simulink model "Vergleich_MRAC"  (Simulink 7.8)
settings: Solver=ode45  StartTime=0.0  StopTime=40  MaxStep=1e-4  RelTol=1e-4
values from neighbouring files (symbols this model uses):
  A = [0,1;-0.4,-0.5]    [Vergleich_MRAC_L1.m]
  Am = [0,1;-2,-2]    [Vergleich_MRAC_L1.m]
  b = [0;1]    [Vergleich_MRAC_L1.m]
  c = [1,0]    [Vergleich_MRAC_L1.m]
  cm = [1,0]    [Vergleich_MRAC_L1.m]
  Gamma2 = 10    [Vergleich_MRAC_L1.m]
  kg = -1/(c*inv(Am)*b)    [Vergleich_MRAC_L1.m]
  km = [1.6,1.5]    [Vergleich_MRAC_L1.m]
  Pb = P*b    [Vergleich_MRAC_L1.m]
  theta = [1,-1]    [Vergleich_MRAC_L1.m]
libraries: simulink x1
settings Model: Creator=Markus  LastModifiedBy=Markus

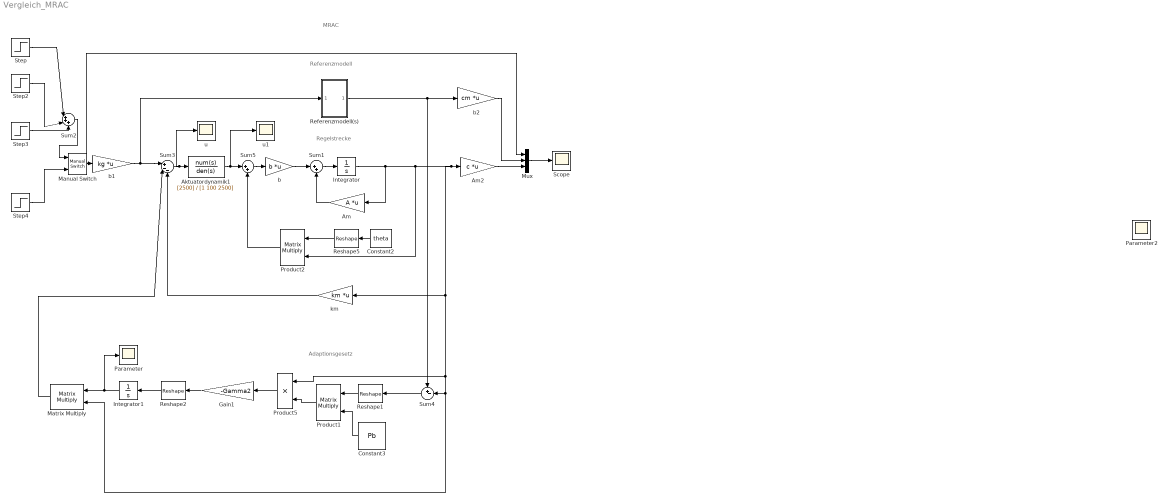
== system Vergleich_MRAC ==
  note: Regelstrecke
  note: Adaptionsgesetz
  note: Referenzmodell
  note: MRAC
  Aktuatordynamik1 : TransferFcn  Numerator=[2500]  Denominator=[1 100 2500]
  Am : Gain  Gain=A  Multiplication=Matrix(K*u)
  Am2 : Gain  Gain=c  Multiplication=Matrix(K*u)
  Constant2 : Constant  Value=theta
  Constant3 : Constant  Value=Pb
  Gain1 : Gain  Gain=-Gamma2
  Integrator : Integrator
  Integrator1 : Integrator
  Manual Switch : simulink/Signal Routing/Manual Switch  sw=1  action=0  varsize=off
  Matrix Multiply : Product  Multiplication=Matrix(*)
  Mux : Mux  Inputs=3
  Parameter : Scope
      settings: TimeRange=40  YMin=-1.4  YMax=0  SaveName=simout
  Parameter2 : Scope
      settings: TimeRange=15  YMin=-1  SaveName=ScopeData13
  Product1 : Product  Multiplication=Matrix(*)  RndMeth=Zero
  Product2 : Product  Multiplication=Matrix(*)  RndMeth=Zero
  Product5 : Product  RndMeth=Zero
  Referenzmodell(s) : Subsystem
  Reshape1 : Reshape  OutputDimensionality=Row vector (2-D)
  Reshape2 : Reshape  OutputDimensionality=Row vector (2-D)
  Reshape5 : Reshape  OutputDimensionality=Row vector (2-D)
  Scope : Scope
      settings: TimeRange=15  YMin=1.9  YMax=4.2  SaveName=Sim_data4  DataFormat=Array
  Step : Step  SampleTime=0
  Step2 : Step  Time=11  SampleTime=0
  Step3 : Step  Time=21  After=2  SampleTime=0
  Step4 : Step  SampleTime=0
  Sum1 : Sum  Inputs=|++
  Sum2 : Sum  Inputs=|+++
  Sum3 : Sum  Inputs=|+--
  Sum4 : Sum  Inputs=+-|
  Sum5 : Sum  Inputs=|++
  b : Gain  Gain=b  Multiplication=Matrix(K*u)
  b1 : Gain  Gain=kg  Multiplication=Matrix(K*u)
  b2 : Gain  Gain=cm  Multiplication=Matrix(K*u)
  km : Gain  Gain=km  Multiplication=Matrix(K*u)
  u : Scope
      settings: TimeRange=20  YMin=2.75  YMax=7  SaveName=ScopeData2
  u1 : Scope
      settings: TimeRange=20  YMin=2.75  YMax=7
  wires:
  Integrator/1 -> Am/1, Am2/1, Product5/1, Sum4/2, Matrix Multiply/2, km/1, Product2/2
  Sum1/1 -> Integrator/1
  b/1 -> Sum1/1
  Constant2/1 -> Reshape5/1
  Reshape5/1 -> Product2/1
  Am2/1 -> Mux/3
  Mux/1 -> Scope/1
  Am/1 -> Sum1/2
  Manual Switch/1 -> b1/1, Mux/1
  b1/1 -> Referenzmodell(s)/1(In1), Sum3/1
  b2/1 -> Mux/2
  Referenzmodell(s)/1(Out1) -> b2/1, Sum4/1
  Sum4/1 -> Reshape1/1
  Constant3/1 -> Product1/2
  Reshape1/1 -> Product1/1
  Product1/1 -> Product5/2
  Product5/1 -> Gain1/1
  Gain1/1 -> Reshape2/1
  Reshape2/1 -> Integrator1/1
  Sum5/1 -> b/1
  km/1 -> Sum3/3
  ? -> Parameter2/1
  Sum2/1 -> Manual Switch/1
  Matrix Multiply/1 -> Sum3/2
  Integrator1/1 -> Matrix Multiply/1, Parameter/1
  Sum3/1 -> Aktuatordynamik1/1, u/1
  Product2/1 -> Sum5/2
  Step/1 -> Sum2/1
  Step4/1 -> Manual Switch/2
  Aktuatordynamik1/1 -> Sum5/1, u1/1
  Step2/1 -> Sum2/2
  Step3/1 -> Sum2/3

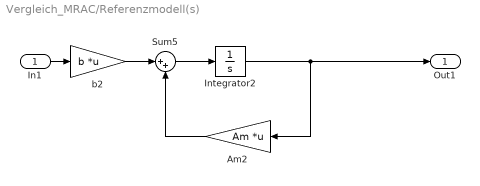
== system Vergleich_MRAC/Referenzmodell(s) ==
  In1 : Inport  PortDimensions=[1,1]
  Am2 : Gain  Gain=Am  Multiplication=Matrix(K*u)
  Integrator2 : Integrator
  Sum5 : Sum  Inputs=|++
  b2 : Gain  Gain=b  Multiplication=Matrix(K*u)
  Out1 : Outport
  wires:
  Integrator2/1 -> Am2/1, Out1/1
  Sum5/1 -> Integrator2/1
  b2/1 -> Sum5/1
  Am2/1 -> Sum5/2
  In1/1 -> b2/1
